simulink model "sim_test"  (R2022a)
settings: Solver=VariableStepAuto  StartTime=0.0  StopTime=10.0  RelTol=1e-3
settings Model: Creator=gleam  LastModifiedBy=gleam

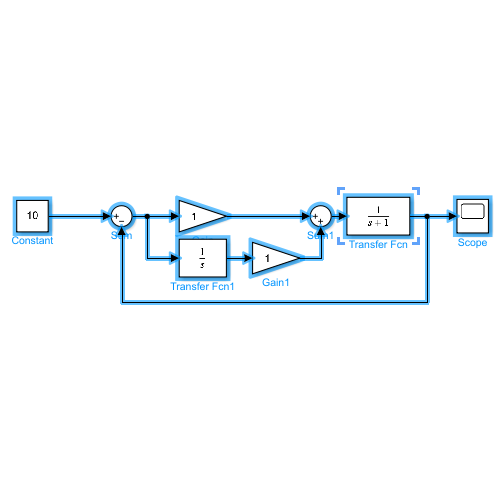
[thumbnail: Simulink's stored preview of the top-level diagram]
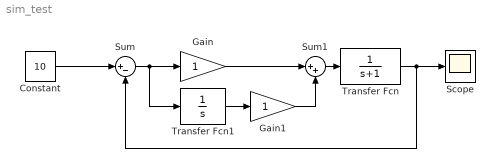
== system sim_test ==
  Constant : Constant  Value=10
  Gain : Gain
  Gain1 : Gain
  Scope : Scope
  Sum : Sum  Inputs=|+-
  Sum1 : Sum  Inputs=|++
  Transfer Fcn : TransferFcn  Denominator=[1 1]
  Transfer Fcn1 : TransferFcn  Denominator=[1 0]
  wires:
  Constant/1 -> Sum/1
  Sum/1 -> Transfer Fcn1/1, Gain/1
  Gain/1 -> Sum1/1
  Transfer Fcn/1 -> Sum/2, Scope/1
  Transfer Fcn1/1 -> Gain1/1
  Sum1/1 -> Transfer Fcn/1
  Gain1/1 -> Sum1/2
